simulink model "gm_untitled"  (R2022a)
settings: Solver=FixedStepDiscrete  StartTime=0.0  StopTime=2000  RelTol=1e-3
libraries: dspsigops x3, simulink x1, hdlsllib x1, simulink_need_slupdate x1
Description:
  | Symmetric FIR Filter
  | This example shows how to use HDL Coder(TM) to check, generate,
  | and verify HDL for a fixed-point symmetric FIR filter.
settings Model: Creator=okoko  LastModifiedBy=okoko
settings SolverCC: AlgebraicLoopSolver=TrustRegion
settings DataIOCC: LimitDataPoints=on  SaveOutput=off  SignalLogging=off  SaveTime=off  SignalLoggingName=logsOut
settings OptimizationCC: BlockReduction=off  BooleanDataType=off  ConditionallyExecuteInputs=off  DefaultParameterBehavior=Inlined  InlineInvariantSignals=on  ExpressionDepthLimit=2147483647  InitFltsAndDblsToZero=on  LifeSpan=inf  BufferReusableBoundary=off
settings DebuggingCC: AlgebraicLoopMsg=error  SaveWithParameterizedLinksMsg=none  UnderspecifiedInitializationDetection=Classic  MergeDetectMultiDrivingBlocksExec=none  CheckExecutionContextPreStartOutputMsg=on  SignalResolutionControl=TryResolveAllWithWarning  InheritedTsInSrcMsg=none  MultiTaskDSMMsg=warning  MultiTaskCondExecSysMsg=none  SingleTaskRateTransMsg=error  IntegerOverflowMsg=none  ParameterPrecisionLossMsg=none  FcnCallInpInsideContextMsg=warning  UnconnectedInputMsg=warning  UnconnectedOutputMsg=warning  UnconnectedLineMsg=warning  BusObjectLabelMismatch=none  AllowSymbolicDim=off  StateNameClashWarn=warning  StrictBusMsg=ErrorOnBusTreatedAsVector  SFUnexpectedBacktrackingDiag=warning  SFNoUnconditionalDefaultTransitionDiag=warning  SFExecutionAtInitializationDiag=none  SFMachineParentedDataDiag=warning  IntegerSaturationMsg=none  ArithmeticOperatorsInVariantConditions=warning
settings HardwareCC: ProdBitPerPointer=32  ProdBitPerSizeT=32  ProdBitPerPtrDiffT=32  ProdLargestAtomicFloat=None  ProdIntDivRoundTo=Undefined  ProdEndianess=Unspecified  ProdWordSize=32  ProdHWDeviceType=ASIC/FPGA->ASIC/FPGA  TargetUnknown=on  ProdEqTarget=off
settings SFSimCC: SimUseLocalCustomCode=off  CustomCodeUndefinedFunction=UseInterfaceOnly
settings RTWCC: RTWUseLocalCustomCode=off
settings CodeAppCC: StateflowObjectComments=on
settings GRTTargetCC: TargetFcnLib=ansi_tfl_tmw.mat  TargetLangStandard=C89/C90 (ANSI)  CombineOutputUpdateFcns=off  GRTInterface=on
settings ConfigComp: CovScope=ReferencedModels  CovMetricSettings=dw  CovSaveCumulativeToWorkspaceVar=on  CovSaveSingleToWorkspaceVar=on  CovExternalEMLEnable=off  CovSFcnEnable=off

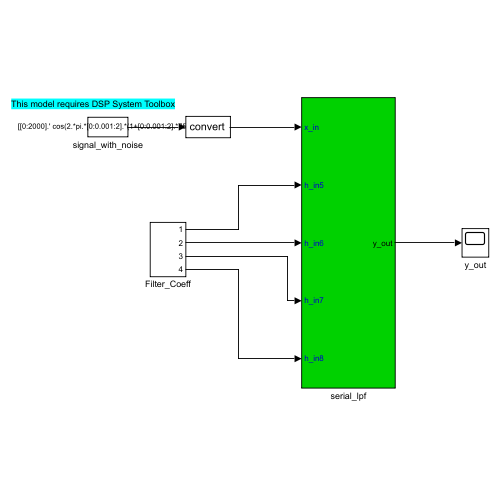
[thumbnail: Simulink's stored preview of the top-level diagram]
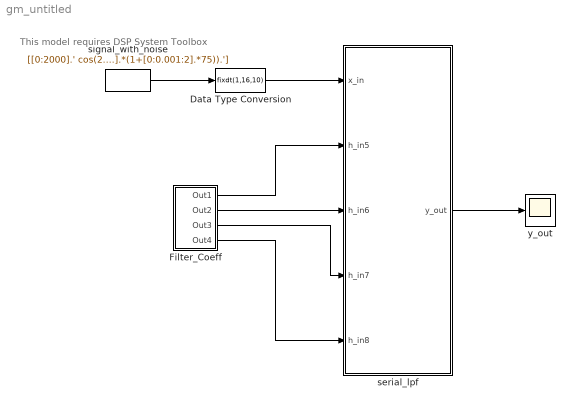
== system gm_untitled ==
  note: This model requires DSP System Toolbox
  Data Type Conversion : DataTypeConversion  OutDataTypeStr=fixdt(1,16,10)  SaturateOnIntegerOverflow=off  RndMeth=Floor
  Filter_Coeff : Subsystem
  serial_lpf : Subsystem
  signal_with_noise : FromWorkspace  VariableName=[[0:2000].' cos(2.*pi.*[0:0.001:2].*(1+[0:0.001:2].*75)).']  SampleTime=1  OutputAfterFinalValue=Setting to zero
  y_out : Scope
  wires:
  Filter_Coeff/4(Out4) -> serial_lpf/5(h_in8)
  Filter_Coeff/3(Out3) -> serial_lpf/4(h_in7)
  Filter_Coeff/2(Out2) -> serial_lpf/3(h_in6)
  Filter_Coeff/1(Out1) -> serial_lpf/2(h_in5)
  serial_lpf/1(y_out) -> y_out/1
  Data Type Conversion/1 -> serial_lpf/1(x_in)
  signal_with_noise/1 -> Data Type Conversion/1

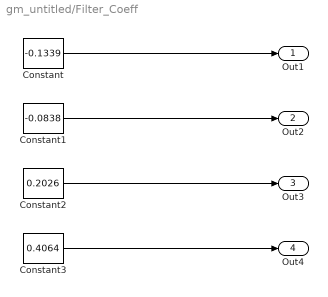
== system gm_untitled/Filter_Coeff ==
  Constant : Constant  Value=-0.1339  OutDataTypeStr=fixdt(1,16,10)  SampleTime=1
  Constant1 : Constant  Value=-0.0838  OutDataTypeStr=fixdt(1,16,10)  SampleTime=1
  Constant2 : Constant  Value=0.2026  OutDataTypeStr=fixdt(1,16,10)  SampleTime=1
  Constant3 : Constant  Value=0.4064  OutDataTypeStr=fixdt(1,16,10)  SampleTime=1
  Out1 : Outport  VectorParamsAs1DForOutWhenUnconnected=off
  Out2 : Outport  Port=2  VectorParamsAs1DForOutWhenUnconnected=off
  Out3 : Outport  Port=3  VectorParamsAs1DForOutWhenUnconnected=off
  Out4 : Outport  Port=4  VectorParamsAs1DForOutWhenUnconnected=off
  wires:
  Constant/1 -> Out1/1
  Constant2/1 -> Out3/1
  Constant3/1 -> Out4/1
  Constant1/1 -> Out2/1

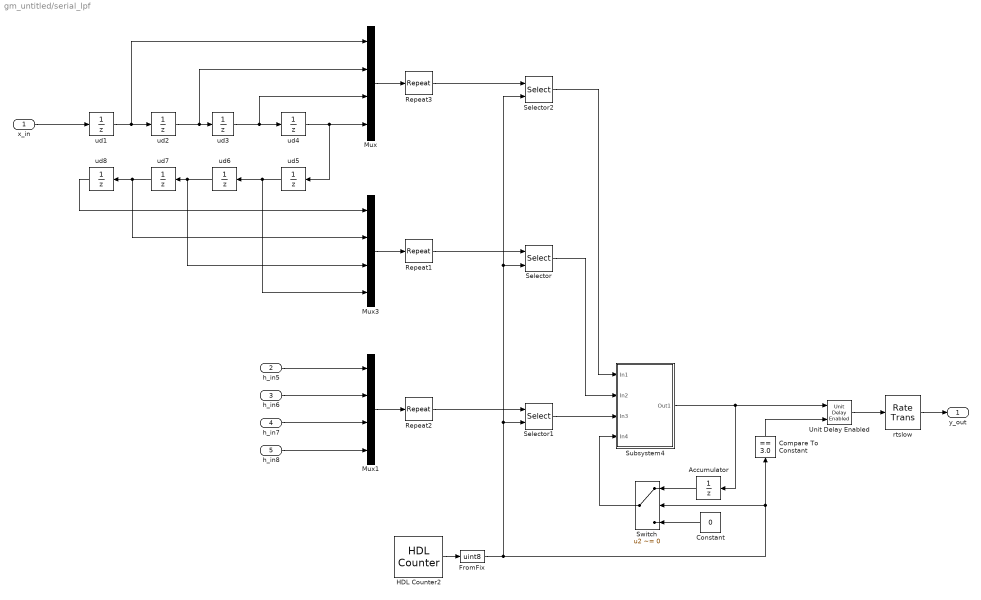
== system gm_untitled/serial_lpf ==
  x_in : Inport  SampleTime=1
  h_in5 : Inport  Port=2
  h_in6 : Inport  Port=3
  h_in7 : Inport  Port=4
  h_in8 : Inport  Port=5
  Accumulator : UnitDelay  SampleTime=-1  HasFrameUpgradeWarning=on
  Compare To Constant : simulink/Logic and Bit Operations/Compare To Constant  relop===  const=3.0  OutDataTypeStr=boolean
  Constant : Constant  Value=0  OutDataTypeStr=Inherit: Inherit via back propagation  SampleTime=-1
  FromFix : DataTypeConversion  OutDataTypeStr=uint8  SaturateOnIntegerOverflow=off  RndMeth=Floor
  HDL Counter2 : hdlsllib/Sources/HDL Counter  CountType=Count limited  CountInit=0  CountStep=1  CountMax=3  CountFromType=Initial value  CountFrom=0  CountResetPort=off  CountLoadPort=off  CountEnbPort=off  CountDirPort=off  CountHitOutputPort=off  CountDataType=Unsigned  CountWordLen=2  CountFracLen=0  CountSampTime=-1
  Mux : Mux
  Mux1 : Mux
  Mux3 : Mux
  Repeat1 : dspsigops/Repeat  N=4  RateOptions=Allow multirate processing  ic=0  mode=Unused parameter value
  Repeat2 : dspsigops/Repeat  N=4  RateOptions=Allow multirate processing  ic=0  mode=Unused parameter value
  Repeat3 : dspsigops/Repeat  N=4  RateOptions=Allow multirate processing  ic=0  mode=Unused parameter value
  Selector : Selector  IndexMode=Zero-based  InputPortWidth=4  IndexOptions=Index vector (port)  Indices=[1 3]  OutputSizes=1
  Selector1 : Selector  IndexMode=Zero-based  InputPortWidth=4  IndexOptions=Index vector (port)  Indices=[1 3]  OutputSizes=1
  Selector2 : Selector  IndexMode=Zero-based  InputPortWidth=4  IndexOptions=Index vector (port)  Indices=[1 3]  OutputSizes=1
  Subsystem4 : Subsystem  TreatAsAtomicUnit=on
  Switch : Switch  Criteria=u2 ~= 0  OutDataTypeStr=fixdt(1,35,20)  SaturateOnIntegerOverflow=off  InputSameDT=off
  Unit Delay Enabled : simulink_need_slupdate/Unit Delay Enabled  vinit=0.0  tsamp=-1
      settings: SourceProductBaseCode=SL
  rtslow : RateTransition
  ud{1..8} (8 alike) : UnitDelay  SampleTime=-1  HasFrameUpgradeWarning=on
  y_out : Outport  SampleTime=1  VectorParamsAs1DForOutWhenUnconnected=off
  wires:
  FromFix/1 -> Compare To Constant/1, Switch/2, Selector2/2, Selector/2, Selector1/2
  ud8/1 -> Mux3/1
  ud6/1 -> ud7/1, Mux3/3
  ud5/1 -> ud6/1, Mux3/4
  ud4/1 -> ud5/1, Mux/4
  ud3/1 -> ud4/1, Mux/3
  ud2/1 -> ud3/1, Mux/2
  ud1/1 -> ud2/1, Mux/1
  Compare To Constant/1 -> Unit Delay Enabled/2
  Switch/1 -> Subsystem4/4(In4)
  Constant/1 -> Switch/3
  Accumulator/1 -> Switch/1
  Unit Delay Enabled/1 -> rtslow/1
  rtslow/1 -> y_out/1
  Repeat2/1 -> Selector1/1
  Repeat3/1 -> Selector2/1
  Mux3/1 -> Repeat1/1
  Selector2/1 -> Subsystem4/1(In1)
  Selector1/1 -> Subsystem4/3(In3)
  Mux1/1 -> Repeat2/1
  HDL Counter2/1 -> FromFix/1
  h_in8/1 -> Mux1/4
  h_in7/1 -> Mux1/3
  h_in6/1 -> Mux1/2
  h_in5/1 -> Mux1/1
  ud7/1 -> ud8/1, Mux3/2
  x_in/1 -> ud1/1
  Subsystem4/1(Out1) -> Unit Delay Enabled/1, Accumulator/1
  Repeat1/1 -> Selector/1
  Mux/1 -> Repeat3/1
  Selector/1 -> Subsystem4/2(In2)

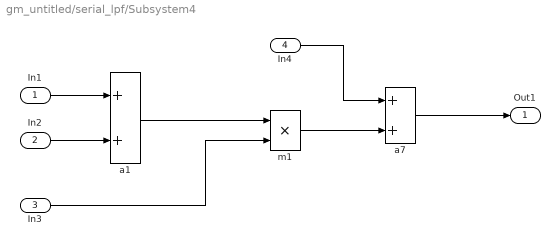
== system gm_untitled/serial_lpf/Subsystem4 ==
  In1 : Inport
  In2 : Inport  Port=2
  In3 : Inport  Port=3
  In4 : Inport  Port=4
  a1 : Sum
  a7 : Sum
  m1 : Product  RndMeth=Zero
  Out1 : Outport  OutDataTypeStr=fixdt(1,35,20)  SampleTime=0.25  VectorParamsAs1DForOutWhenUnconnected=off
  wires:
  m1/1 -> a7/2
  In4/1 -> a7/1
  In3/1 -> m1/2
  In2/1 -> a1/2
  In1/1 -> a1/1
  a7/1 -> Out1/1
  a1/1 -> m1/1
